simulink model "TCS_autosar_arch"  (R2019b)
settings: Solver=VariableStepAuto  StartTime=0.0  StopTime=10.0  RelTol=1e-3
settings Model: Creator=12045  LastModifiedBy=12045

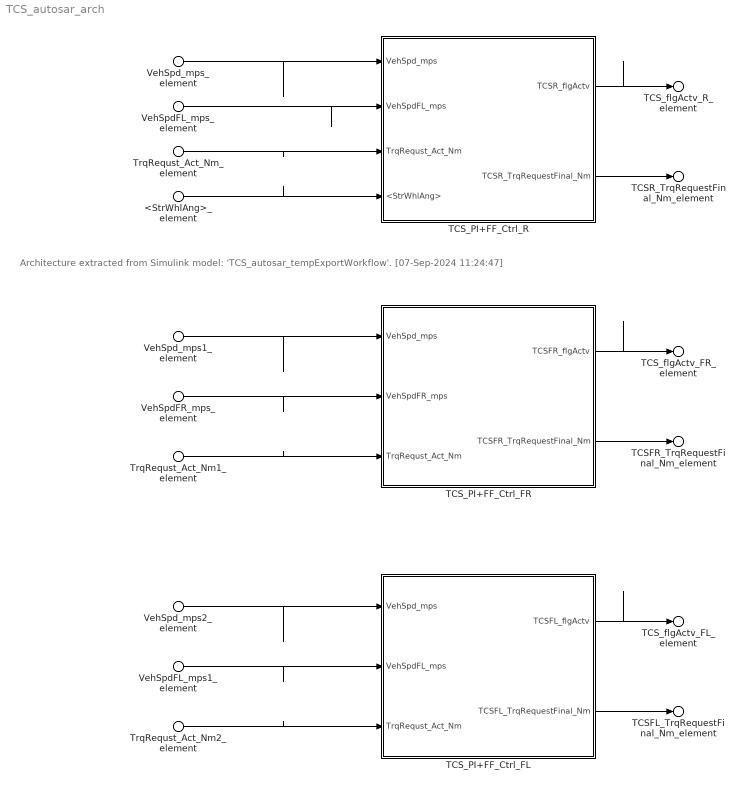
== system TCS_autosar_arch ==
  note: Architecture extracted from Simulink model: 'TCS_autosar_tempExportWorkflow'. [07-Sep-2024 11:24:47]
  VehSpd_mps_element : Inport  PortName=VehSpd_mps
  VehSpdFL_mps_element : Inport  Port=2  PortName=VehSpdFL_mps
  TrqRequst_Act_Nm_element : Inport  Port=3  PortName=TrqRequst_Act_Nm
  <StrWhlAng>_element : Inport  Port=4  PortName=<StrWhlAng>
  VehSpd_mps1_element : Inport  Port=5  PortName=VehSpd_mps1
  VehSpdFR_mps_element : Inport  Port=6  PortName=VehSpdFR_mps
  TrqRequst_Act_Nm1_element : Inport  Port=7  PortName=TrqRequst_Act_Nm1
  VehSpd_mps2_element : Inport  Port=8  PortName=VehSpd_mps2
  VehSpdFL_mps1_element : Inport  Port=9  PortName=VehSpdFL_mps1
  TrqRequst_Act_Nm2_element : Inport  Port=10  PortName=TrqRequst_Act_Nm2
  TCS_PI+FF_Ctrl_FL : Subsystem
      settings: PortSchema="{\"entries\":[{\"content\":{\"headerSize\":26,\"margin\":15,\"minimumSpacing\":25,\"sides\":[{\"content\":{\"connectorIds\":[\"In1\",\"In2\",\"In3\"]},\"type\":\"ConnectorPlacement.EquallySpacedRectSide\",\"uuid\":\"eaf1fc9b-c735-4d64-9f98-dd2769dd9966\"},{\"content\":{\"connectorIds\":[\"Out1\",\"Out2\"],\"side\":\"RIGHT\"},\"type\":\"ConnectorPlacement.EquallySpacedRectSide\",\"uuid\":\"44921fe4-cdee-42c2-ba14-46e851cbb056\"},{\"content\":{\"connectorIds\":[],\"side\":\"TOP\"},\"type\":\"ConnectorPlacement.EquallySpacedRectSide\",\"uuid\":\"3b219d8e-8c01-443b-b35e-1f0c6839a481\"}]},\"type\":\"ConnectorPlacement.EquallySpacedConnector\",\"uuid\":\"03372050-c4f7-4141-ad1c-5172546441aa\"}],\"packageUris\":[\"http://schema.mathworks.com/mf0/Connector/19700101\"],\"version\":\"1.0\"}"
  TCS_PI+FF_Ctrl_FR : Subsystem
      settings: PortSchema="{\"entries\":[{\"content\":{\"headerSize\":26,\"margin\":15,\"minimumSpacing\":25,\"sides\":[{\"content\":{\"connectorIds\":[\"In1\",\"In2\",\"In3\"]},\"type\":\"ConnectorPlacement.EquallySpacedRectSide\",\"uuid\":\"eaf1fc9b-c735-4d64-9f98-dd2769dd9966\"},{\"content\":{\"connectorIds\":[\"Out1\",\"Out2\"],\"side\":\"RIGHT\"},\"type\":\"ConnectorPlacement.EquallySpacedRectSide\",\"uuid\":\"44921fe4-cdee-42c2-ba14-46e851cbb056\"},{\"content\":{\"connectorIds\":[],\"side\":\"TOP\"},\"type\":\"ConnectorPlacement.EquallySpacedRectSide\",\"uuid\":\"3b219d8e-8c01-443b-b35e-1f0c6839a481\"}]},\"type\":\"ConnectorPlacement.EquallySpacedConnector\",\"uuid\":\"03372050-c4f7-4141-ad1c-5172546441aa\"}],\"packageUris\":[\"http://schema.mathworks.com/mf0/Connector/19700101\"],\"version\":\"1.0\"}"
  TCS_PI+FF_Ctrl_R : Subsystem
      settings: PortSchema="{\"entries\":[{\"content\":{\"headerSize\":26,\"margin\":15,\"minimumSpacing\":25,\"sides\":[{\"content\":{\"connectorIds\":[\"In1\",\"In2\",\"In3\",\"In4\"]},\"type\":\"ConnectorPlacement.EquallySpacedRectSide\",\"uuid\":\"eaf1fc9b-c735-4d64-9f98-dd2769dd9966\"},{\"content\":{\"connectorIds\":[\"Out1\",\"Out2\"],\"side\":\"RIGHT\"},\"type\":\"ConnectorPlacement.EquallySpacedRectSide\",\"uuid\":\"44921fe4-cdee-42c2-ba14-46e851cbb056\"},{\"content\":{\"connectorIds\":[],\"side\":\"TOP\"},\"type\":\"ConnectorPlacement.EquallySpacedRectSide\",\"uuid\":\"3b219d8e-8c01-443b-b35e-1f0c6839a481\"}]},\"type\":\"ConnectorPlacement.EquallySpacedConnector\",\"uuid\":\"03372050-c4f7-4141-ad1c-5172546441aa\"}],\"packageUris\":[\"http://schema.mathworks.com/mf0/Connector/19700101\"],\"version\":\"1.0\"}"
  TCS_flgActv_R_element : Outport  PortName=TCS_flgActv_R
  TCSR_TrqRequestFinal_Nm_element : Outport  Port=2  PortName=TCSR_TrqRequestFinal_Nm
  TCS_flgActv_FR_element : Outport  Port=3  PortName=TCS_flgActv_FR
  TCSFR_TrqRequestFinal_Nm_element : Outport  Port=4  PortName=TCSFR_TrqRequestFinal_Nm
  TCS_flgActv_FL_element : Outport  Port=5  PortName=TCS_flgActv_FL
  TCSFL_TrqRequestFinal_Nm_element : Outport  Port=6  PortName=TCSFL_TrqRequestFinal_Nm
  wires:
  VehSpd_mps2_element/1 -> TCS_PI+FF_Ctrl_FL/1(VehSpd_mps)
  VehSpdFL_mps1_element/1 -> TCS_PI+FF_Ctrl_FL/2(VehSpdFL_mps)
  TrqRequst_Act_Nm2_element/1 -> TCS_PI+FF_Ctrl_FL/3(TrqRequst_Act_Nm)
  VehSpd_mps1_element/1 -> TCS_PI+FF_Ctrl_FR/1(VehSpd_mps)
  VehSpdFR_mps_element/1 -> TCS_PI+FF_Ctrl_FR/2(VehSpdFR_mps)
  TrqRequst_Act_Nm1_element/1 -> TCS_PI+FF_Ctrl_FR/3(TrqRequst_Act_Nm)
  VehSpd_mps_element/1 -> TCS_PI+FF_Ctrl_R/1(VehSpd_mps)
  VehSpdFL_mps_element/1 -> TCS_PI+FF_Ctrl_R/2(VehSpdFL_mps)
  TrqRequst_Act_Nm_element/1 -> TCS_PI+FF_Ctrl_R/3(TrqRequst_Act_Nm)
  <StrWhlAng>_element/1 -> TCS_PI+FF_Ctrl_R/4(<StrWhlAng>)
  TCS_PI+FF_Ctrl_R/1(TCSR_flgActv) -> TCS_flgActv_R_element/1
  TCS_PI+FF_Ctrl_R/2(TCSR_TrqRequestFinal_Nm) -> TCSR_TrqRequestFinal_Nm_element/1
  TCS_PI+FF_Ctrl_FR/1(TCSFR_flgActv) -> TCS_flgActv_FR_element/1
  TCS_PI+FF_Ctrl_FR/2(TCSFR_TrqRequestFinal_Nm) -> TCSFR_TrqRequestFinal_Nm_element/1
  TCS_PI+FF_Ctrl_FL/1(TCSFL_flgActv) -> TCS_flgActv_FL_element/1
  TCS_PI+FF_Ctrl_FL/2(TCSFL_TrqRequestFinal_Nm) -> TCSFL_TrqRequestFinal_Nm_element/1

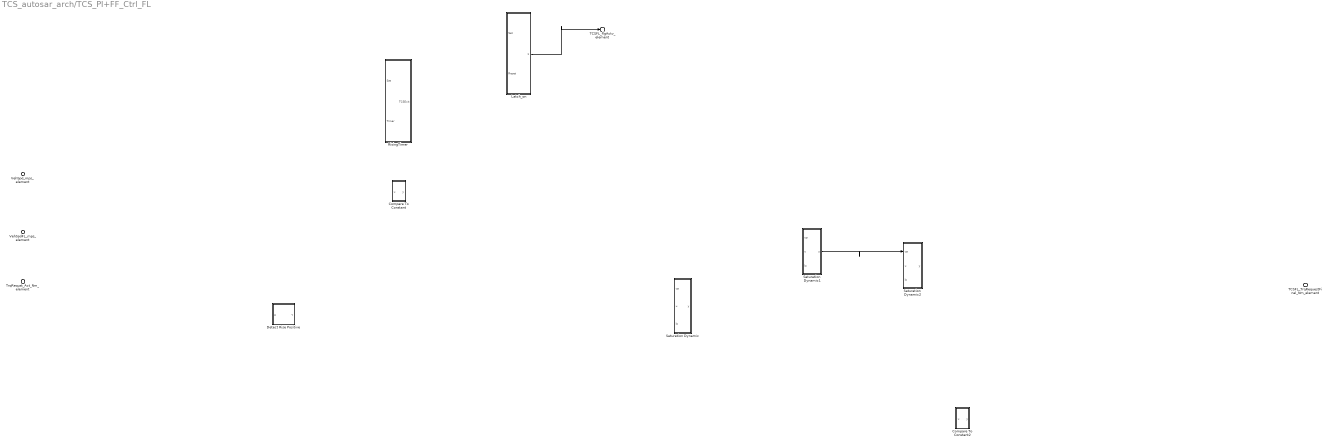
== system TCS_autosar_arch/TCS_PI+FF_Ctrl_FL ==
  VehSpd_mps_element : Inport  PortName=VehSpd_mps
  VehSpdFL_mps_element : Inport  Port=2  PortName=VehSpdFL_mps
  TrqRequst_Act_Nm_element : Inport  Port=3  PortName=TrqRequst_Act_Nm
  Compare To Constant : Subsystem
      settings: PortSchema="{\"entries\":[{\"content\":{\"headerSize\":26,\"margin\":15,\"minimumSpacing\":25,\"sides\":[{\"content\":{\"connectorIds\":[\"In1\"]},\"type\":\"ConnectorPlacement.EquallySpacedRectSide\",\"uuid\":\"eaf1fc9b-c735-4d64-9f98-dd2769dd9966\"},{\"content\":{\"connectorIds\":[\"Out1\"],\"side\":\"RIGHT\"},\"type\":\"ConnectorPlacement.EquallySpacedRectSide\",\"uuid\":\"44921fe4-cdee-42c2-ba14-46e851cbb056\"},{\"content\":{\"connectorIds\":[],\"side\":\"TOP\"},\"type\":\"ConnectorPlacement.EquallySpacedRectSide\",\"uuid\":\"3b219d8e-8c01-443b-b35e-1f0c6839a481\"}]},\"type\":\"ConnectorPlacement.EquallySpacedConnector\",\"uuid\":\"03372050-c4f7-4141-ad1c-5172546441aa\"}],\"packageUris\":[\"http://schema.mathworks.com/mf0/Connector/19700101\"],\"version\":\"1.0\"}"
  Compare To Constant2 : Subsystem
      settings: PortSchema="{\"entries\":[{\"content\":{\"headerSize\":26,\"margin\":15,\"minimumSpacing\":25,\"sides\":[{\"content\":{\"connectorIds\":[\"In1\"]},\"type\":\"ConnectorPlacement.EquallySpacedRectSide\",\"uuid\":\"eaf1fc9b-c735-4d64-9f98-dd2769dd9966\"},{\"content\":{\"connectorIds\":[\"Out1\"],\"side\":\"RIGHT\"},\"type\":\"ConnectorPlacement.EquallySpacedRectSide\",\"uuid\":\"44921fe4-cdee-42c2-ba14-46e851cbb056\"},{\"content\":{\"connectorIds\":[],\"side\":\"TOP\"},\"type\":\"ConnectorPlacement.EquallySpacedRectSide\",\"uuid\":\"3b219d8e-8c01-443b-b35e-1f0c6839a481\"}]},\"type\":\"ConnectorPlacement.EquallySpacedConnector\",\"uuid\":\"03372050-c4f7-4141-ad1c-5172546441aa\"}],\"packageUris\":[\"http://schema.mathworks.com/mf0/Connector/19700101\"],\"version\":\"1.0\"}"
  Detect Rise Positive : Subsystem
      settings: PortSchema="{\"entries\":[{\"content\":{\"headerSize\":26,\"margin\":15,\"minimumSpacing\":25,\"sides\":[{\"content\":{\"connectorIds\":[\"In1\"]},\"type\":\"ConnectorPlacement.EquallySpacedRectSide\",\"uuid\":\"eaf1fc9b-c735-4d64-9f98-dd2769dd9966\"},{\"content\":{\"connectorIds\":[\"Out1\"],\"side\":\"RIGHT\"},\"type\":\"ConnectorPlacement.EquallySpacedRectSide\",\"uuid\":\"44921fe4-cdee-42c2-ba14-46e851cbb056\"},{\"content\":{\"connectorIds\":[],\"side\":\"TOP\"},\"type\":\"ConnectorPlacement.EquallySpacedRectSide\",\"uuid\":\"3b219d8e-8c01-443b-b35e-1f0c6839a481\"}]},\"type\":\"ConnectorPlacement.EquallySpacedConnector\",\"uuid\":\"03372050-c4f7-4141-ad1c-5172546441aa\"}],\"packageUris\":[\"http://schema.mathworks.com/mf0/Connector/19700101\"],\"version\":\"1.0\"}"
  Latch_on : Subsystem
      settings: PortSchema="{\"entries\":[{\"content\":{\"headerSize\":26,\"margin\":15,\"minimumSpacing\":25,\"sides\":[{\"content\":{\"connectorIds\":[\"In1\",\"In2\"]},\"type\":\"ConnectorPlacement.EquallySpacedRectSide\",\"uuid\":\"eaf1fc9b-c735-4d64-9f98-dd2769dd9966\"},{\"content\":{\"connectorIds\":[\"Out1\"],\"side\":\"RIGHT\"},\"type\":\"ConnectorPlacement.EquallySpacedRectSide\",\"uuid\":\"44921fe4-cdee-42c2-ba14-46e851cbb056\"},{\"content\":{\"connectorIds\":[],\"side\":\"TOP\"},\"type\":\"ConnectorPlacement.EquallySpacedRectSide\",\"uuid\":\"3b219d8e-8c01-443b-b35e-1f0c6839a481\"}]},\"type\":\"ConnectorPlacement.EquallySpacedConnector\",\"uuid\":\"03372050-c4f7-4141-ad1c-5172546441aa\"}],\"packageUris\":[\"http://schema.mathworks.com/mf0/Connector/19700101\"],\"version\":\"1.0\"}"
  RisingTimer : Subsystem
      settings: PortSchema="{\"entries\":[{\"content\":{\"headerSize\":26,\"margin\":15,\"minimumSpacing\":25,\"sides\":[{\"content\":{\"connectorIds\":[\"In1\",\"In2\"]},\"type\":\"ConnectorPlacement.EquallySpacedRectSide\",\"uuid\":\"eaf1fc9b-c735-4d64-9f98-dd2769dd9966\"},{\"content\":{\"connectorIds\":[\"Out1\"],\"side\":\"RIGHT\"},\"type\":\"ConnectorPlacement.EquallySpacedRectSide\",\"uuid\":\"44921fe4-cdee-42c2-ba14-46e851cbb056\"},{\"content\":{\"connectorIds\":[],\"side\":\"TOP\"},\"type\":\"ConnectorPlacement.EquallySpacedRectSide\",\"uuid\":\"3b219d8e-8c01-443b-b35e-1f0c6839a481\"}]},\"type\":\"ConnectorPlacement.EquallySpacedConnector\",\"uuid\":\"03372050-c4f7-4141-ad1c-5172546441aa\"}],\"packageUris\":[\"http://schema.mathworks.com/mf0/Connector/19700101\"],\"version\":\"1.0\"}"
  Saturation Dynamic : Subsystem
      settings: PortSchema="{\"entries\":[{\"content\":{\"headerSize\":26,\"margin\":15,\"minimumSpacing\":25,\"sides\":[{\"content\":{\"connectorIds\":[\"In1\",\"In2\",\"In3\"]},\"type\":\"ConnectorPlacement.EquallySpacedRectSide\",\"uuid\":\"eaf1fc9b-c735-4d64-9f98-dd2769dd9966\"},{\"content\":{\"connectorIds\":[\"Out1\"],\"side\":\"RIGHT\"},\"type\":\"ConnectorPlacement.EquallySpacedRectSide\",\"uuid\":\"44921fe4-cdee-42c2-ba14-46e851cbb056\"},{\"content\":{\"connectorIds\":[],\"side\":\"TOP\"},\"type\":\"ConnectorPlacement.EquallySpacedRectSide\",\"uuid\":\"3b219d8e-8c01-443b-b35e-1f0c6839a481\"}]},\"type\":\"ConnectorPlacement.EquallySpacedConnector\",\"uuid\":\"03372050-c4f7-4141-ad1c-5172546441aa\"}],\"packageUris\":[\"http://schema.mathworks.com/mf0/Connector/19700101\"],\"version\":\"1.0\"}"
  Saturation Dynamic1 : Subsystem
      settings: PortSchema="{\"entries\":[{\"content\":{\"headerSize\":26,\"margin\":15,\"minimumSpacing\":25,\"sides\":[{\"content\":{\"connectorIds\":[\"In1\",\"In2\",\"In3\"]},\"type\":\"ConnectorPlacement.EquallySpacedRectSide\",\"uuid\":\"eaf1fc9b-c735-4d64-9f98-dd2769dd9966\"},{\"content\":{\"connectorIds\":[\"Out1\"],\"side\":\"RIGHT\"},\"type\":\"ConnectorPlacement.EquallySpacedRectSide\",\"uuid\":\"44921fe4-cdee-42c2-ba14-46e851cbb056\"},{\"content\":{\"connectorIds\":[],\"side\":\"TOP\"},\"type\":\"ConnectorPlacement.EquallySpacedRectSide\",\"uuid\":\"3b219d8e-8c01-443b-b35e-1f0c6839a481\"}]},\"type\":\"ConnectorPlacement.EquallySpacedConnector\",\"uuid\":\"03372050-c4f7-4141-ad1c-5172546441aa\"}],\"packageUris\":[\"http://schema.mathworks.com/mf0/Connector/19700101\"],\"version\":\"1.0\"}"
  Saturation Dynamic2 : Subsystem
      settings: PortSchema="{\"entries\":[{\"content\":{\"headerSize\":26,\"margin\":15,\"minimumSpacing\":25,\"sides\":[{\"content\":{\"connectorIds\":[\"In1\",\"In2\",\"In3\"]},\"type\":\"ConnectorPlacement.EquallySpacedRectSide\",\"uuid\":\"eaf1fc9b-c735-4d64-9f98-dd2769dd9966\"},{\"content\":{\"connectorIds\":[\"Out1\"],\"side\":\"RIGHT\"},\"type\":\"ConnectorPlacement.EquallySpacedRectSide\",\"uuid\":\"44921fe4-cdee-42c2-ba14-46e851cbb056\"},{\"content\":{\"connectorIds\":[],\"side\":\"TOP\"},\"type\":\"ConnectorPlacement.EquallySpacedRectSide\",\"uuid\":\"3b219d8e-8c01-443b-b35e-1f0c6839a481\"}]},\"type\":\"ConnectorPlacement.EquallySpacedConnector\",\"uuid\":\"03372050-c4f7-4141-ad1c-5172546441aa\"}],\"packageUris\":[\"http://schema.mathworks.com/mf0/Connector/19700101\"],\"version\":\"1.0\"}"
  TCSFL_flgActv_element : Outport  PortName=TCSFL_flgActv
  TCSFL_TrqRequestFinal_Nm_element : Outport  Port=2  PortName=TCSFL_TrqRequestFinal_Nm
  wires:
  Saturation Dynamic1/1(y) -> Saturation Dynamic2/1(up)
  Latch_on/1(flg_TCSActv) -> TCSFL_flgActv_element/1

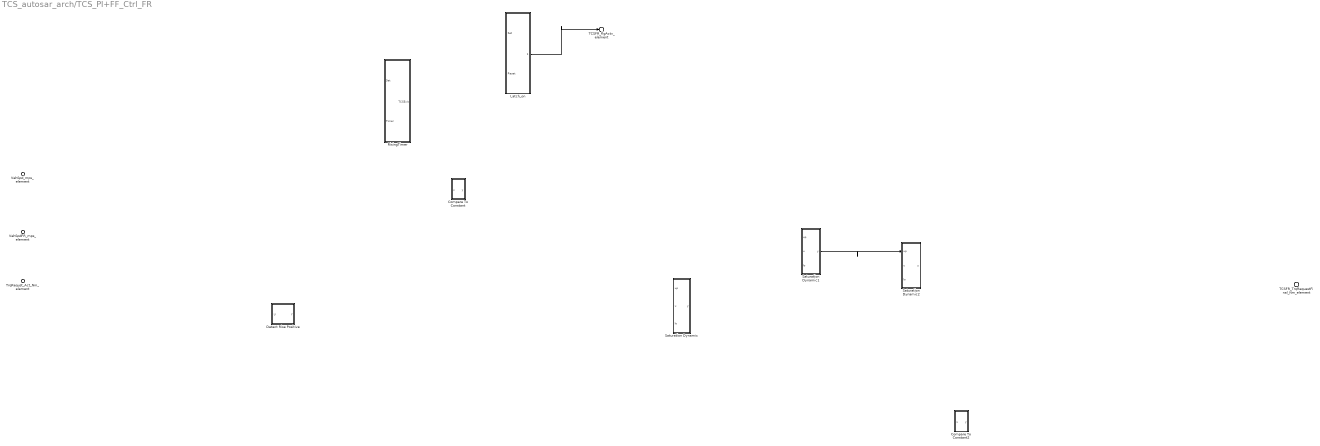
== system TCS_autosar_arch/TCS_PI+FF_Ctrl_FR ==
  VehSpd_mps_element : Inport  PortName=VehSpd_mps
  VehSpdFR_mps_element : Inport  Port=2  PortName=VehSpdFR_mps
  TrqRequst_Act_Nm_element : Inport  Port=3  PortName=TrqRequst_Act_Nm
  Compare To Constant : Subsystem
      settings: PortSchema="{\"entries\":[{\"content\":{\"headerSize\":26,\"margin\":15,\"minimumSpacing\":25,\"sides\":[{\"content\":{\"connectorIds\":[\"In1\"]},\"type\":\"ConnectorPlacement.EquallySpacedRectSide\",\"uuid\":\"eaf1fc9b-c735-4d64-9f98-dd2769dd9966\"},{\"content\":{\"connectorIds\":[\"Out1\"],\"side\":\"RIGHT\"},\"type\":\"ConnectorPlacement.EquallySpacedRectSide\",\"uuid\":\"44921fe4-cdee-42c2-ba14-46e851cbb056\"},{\"content\":{\"connectorIds\":[],\"side\":\"TOP\"},\"type\":\"ConnectorPlacement.EquallySpacedRectSide\",\"uuid\":\"3b219d8e-8c01-443b-b35e-1f0c6839a481\"}]},\"type\":\"ConnectorPlacement.EquallySpacedConnector\",\"uuid\":\"03372050-c4f7-4141-ad1c-5172546441aa\"}],\"packageUris\":[\"http://schema.mathworks.com/mf0/Connector/19700101\"],\"version\":\"1.0\"}"
  Compare To Constant2 : Subsystem
      settings: PortSchema="{\"entries\":[{\"content\":{\"headerSize\":26,\"margin\":15,\"minimumSpacing\":25,\"sides\":[{\"content\":{\"connectorIds\":[\"In1\"]},\"type\":\"ConnectorPlacement.EquallySpacedRectSide\",\"uuid\":\"eaf1fc9b-c735-4d64-9f98-dd2769dd9966\"},{\"content\":{\"connectorIds\":[\"Out1\"],\"side\":\"RIGHT\"},\"type\":\"ConnectorPlacement.EquallySpacedRectSide\",\"uuid\":\"44921fe4-cdee-42c2-ba14-46e851cbb056\"},{\"content\":{\"connectorIds\":[],\"side\":\"TOP\"},\"type\":\"ConnectorPlacement.EquallySpacedRectSide\",\"uuid\":\"3b219d8e-8c01-443b-b35e-1f0c6839a481\"}]},\"type\":\"ConnectorPlacement.EquallySpacedConnector\",\"uuid\":\"03372050-c4f7-4141-ad1c-5172546441aa\"}],\"packageUris\":[\"http://schema.mathworks.com/mf0/Connector/19700101\"],\"version\":\"1.0\"}"
  Detect Rise Positive : Subsystem
      settings: PortSchema="{\"entries\":[{\"content\":{\"headerSize\":26,\"margin\":15,\"minimumSpacing\":25,\"sides\":[{\"content\":{\"connectorIds\":[\"In1\"]},\"type\":\"ConnectorPlacement.EquallySpacedRectSide\",\"uuid\":\"eaf1fc9b-c735-4d64-9f98-dd2769dd9966\"},{\"content\":{\"connectorIds\":[\"Out1\"],\"side\":\"RIGHT\"},\"type\":\"ConnectorPlacement.EquallySpacedRectSide\",\"uuid\":\"44921fe4-cdee-42c2-ba14-46e851cbb056\"},{\"content\":{\"connectorIds\":[],\"side\":\"TOP\"},\"type\":\"ConnectorPlacement.EquallySpacedRectSide\",\"uuid\":\"3b219d8e-8c01-443b-b35e-1f0c6839a481\"}]},\"type\":\"ConnectorPlacement.EquallySpacedConnector\",\"uuid\":\"03372050-c4f7-4141-ad1c-5172546441aa\"}],\"packageUris\":[\"http://schema.mathworks.com/mf0/Connector/19700101\"],\"version\":\"1.0\"}"
  Latch_on : Subsystem
      settings: PortSchema="{\"entries\":[{\"content\":{\"headerSize\":26,\"margin\":15,\"minimumSpacing\":25,\"sides\":[{\"content\":{\"connectorIds\":[\"In1\",\"In2\"]},\"type\":\"ConnectorPlacement.EquallySpacedRectSide\",\"uuid\":\"eaf1fc9b-c735-4d64-9f98-dd2769dd9966\"},{\"content\":{\"connectorIds\":[\"Out1\"],\"side\":\"RIGHT\"},\"type\":\"ConnectorPlacement.EquallySpacedRectSide\",\"uuid\":\"44921fe4-cdee-42c2-ba14-46e851cbb056\"},{\"content\":{\"connectorIds\":[],\"side\":\"TOP\"},\"type\":\"ConnectorPlacement.EquallySpacedRectSide\",\"uuid\":\"3b219d8e-8c01-443b-b35e-1f0c6839a481\"}]},\"type\":\"ConnectorPlacement.EquallySpacedConnector\",\"uuid\":\"03372050-c4f7-4141-ad1c-5172546441aa\"}],\"packageUris\":[\"http://schema.mathworks.com/mf0/Connector/19700101\"],\"version\":\"1.0\"}"
  RisingTimer : Subsystem
      settings: PortSchema="{\"entries\":[{\"content\":{\"headerSize\":26,\"margin\":15,\"minimumSpacing\":25,\"sides\":[{\"content\":{\"connectorIds\":[\"In1\",\"In2\"]},\"type\":\"ConnectorPlacement.EquallySpacedRectSide\",\"uuid\":\"eaf1fc9b-c735-4d64-9f98-dd2769dd9966\"},{\"content\":{\"connectorIds\":[\"Out1\"],\"side\":\"RIGHT\"},\"type\":\"ConnectorPlacement.EquallySpacedRectSide\",\"uuid\":\"44921fe4-cdee-42c2-ba14-46e851cbb056\"},{\"content\":{\"connectorIds\":[],\"side\":\"TOP\"},\"type\":\"ConnectorPlacement.EquallySpacedRectSide\",\"uuid\":\"3b219d8e-8c01-443b-b35e-1f0c6839a481\"}]},\"type\":\"ConnectorPlacement.EquallySpacedConnector\",\"uuid\":\"03372050-c4f7-4141-ad1c-5172546441aa\"}],\"packageUris\":[\"http://schema.mathworks.com/mf0/Connector/19700101\"],\"version\":\"1.0\"}"
  Saturation Dynamic : Subsystem
      settings: PortSchema="{\"entries\":[{\"content\":{\"headerSize\":26,\"margin\":15,\"minimumSpacing\":25,\"sides\":[{\"content\":{\"connectorIds\":[\"In1\",\"In2\",\"In3\"]},\"type\":\"ConnectorPlacement.EquallySpacedRectSide\",\"uuid\":\"eaf1fc9b-c735-4d64-9f98-dd2769dd9966\"},{\"content\":{\"connectorIds\":[\"Out1\"],\"side\":\"RIGHT\"},\"type\":\"ConnectorPlacement.EquallySpacedRectSide\",\"uuid\":\"44921fe4-cdee-42c2-ba14-46e851cbb056\"},{\"content\":{\"connectorIds\":[],\"side\":\"TOP\"},\"type\":\"ConnectorPlacement.EquallySpacedRectSide\",\"uuid\":\"3b219d8e-8c01-443b-b35e-1f0c6839a481\"}]},\"type\":\"ConnectorPlacement.EquallySpacedConnector\",\"uuid\":\"03372050-c4f7-4141-ad1c-5172546441aa\"}],\"packageUris\":[\"http://schema.mathworks.com/mf0/Connector/19700101\"],\"version\":\"1.0\"}"
  Saturation Dynamic1 : Subsystem
      settings: PortSchema="{\"entries\":[{\"content\":{\"headerSize\":26,\"margin\":15,\"minimumSpacing\":25,\"sides\":[{\"content\":{\"connectorIds\":[\"In1\",\"In2\",\"In3\"]},\"type\":\"ConnectorPlacement.EquallySpacedRectSide\",\"uuid\":\"eaf1fc9b-c735-4d64-9f98-dd2769dd9966\"},{\"content\":{\"connectorIds\":[\"Out1\"],\"side\":\"RIGHT\"},\"type\":\"ConnectorPlacement.EquallySpacedRectSide\",\"uuid\":\"44921fe4-cdee-42c2-ba14-46e851cbb056\"},{\"content\":{\"connectorIds\":[],\"side\":\"TOP\"},\"type\":\"ConnectorPlacement.EquallySpacedRectSide\",\"uuid\":\"3b219d8e-8c01-443b-b35e-1f0c6839a481\"}]},\"type\":\"ConnectorPlacement.EquallySpacedConnector\",\"uuid\":\"03372050-c4f7-4141-ad1c-5172546441aa\"}],\"packageUris\":[\"http://schema.mathworks.com/mf0/Connector/19700101\"],\"version\":\"1.0\"}"
  Saturation Dynamic2 : Subsystem
      settings: PortSchema="{\"entries\":[{\"content\":{\"headerSize\":26,\"margin\":15,\"minimumSpacing\":25,\"sides\":[{\"content\":{\"connectorIds\":[\"In1\",\"In2\",\"In3\"]},\"type\":\"ConnectorPlacement.EquallySpacedRectSide\",\"uuid\":\"eaf1fc9b-c735-4d64-9f98-dd2769dd9966\"},{\"content\":{\"connectorIds\":[\"Out1\"],\"side\":\"RIGHT\"},\"type\":\"ConnectorPlacement.EquallySpacedRectSide\",\"uuid\":\"44921fe4-cdee-42c2-ba14-46e851cbb056\"},{\"content\":{\"connectorIds\":[],\"side\":\"TOP\"},\"type\":\"ConnectorPlacement.EquallySpacedRectSide\",\"uuid\":\"3b219d8e-8c01-443b-b35e-1f0c6839a481\"}]},\"type\":\"ConnectorPlacement.EquallySpacedConnector\",\"uuid\":\"03372050-c4f7-4141-ad1c-5172546441aa\"}],\"packageUris\":[\"http://schema.mathworks.com/mf0/Connector/19700101\"],\"version\":\"1.0\"}"
  TCSFR_flgActv_element : Outport  PortName=TCSFR_flgActv
  TCSFR_TrqRequestFinal_Nm_element : Outport  Port=2  PortName=TCSFR_TrqRequestFinal_Nm
  wires:
  Saturation Dynamic1/1(y) -> Saturation Dynamic2/1(up)
  Latch_on/1(flg_TCSActv) -> TCSFR_flgActv_element/1

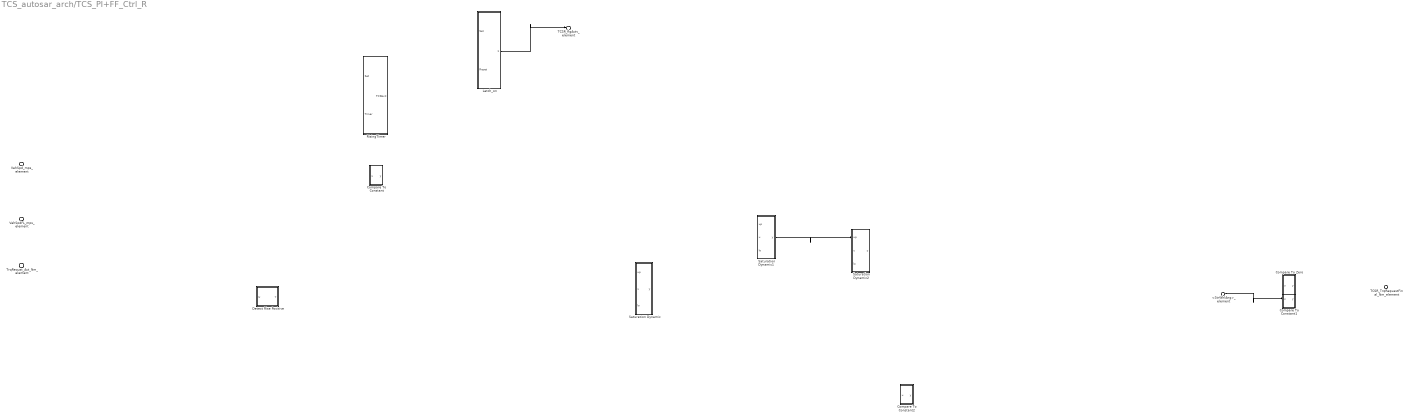
== system TCS_autosar_arch/TCS_PI+FF_Ctrl_R ==
  VehSpd_mps_element : Inport  PortName=VehSpd_mps
  VehSpdFL_mps_element : Inport  Port=2  PortName=VehSpdFL_mps
  TrqRequst_Act_Nm_element : Inport  Port=3  PortName=TrqRequst_Act_Nm
  <StrWhlAng>_element : Inport  Port=4  PortName=<StrWhlAng>
  Compare To Constant : Subsystem
      settings: PortSchema="{\"entries\":[{\"content\":{\"headerSize\":26,\"margin\":15,\"minimumSpacing\":25,\"sides\":[{\"content\":{\"connectorIds\":[\"In1\"]},\"type\":\"ConnectorPlacement.EquallySpacedRectSide\",\"uuid\":\"eaf1fc9b-c735-4d64-9f98-dd2769dd9966\"},{\"content\":{\"connectorIds\":[\"Out1\"],\"side\":\"RIGHT\"},\"type\":\"ConnectorPlacement.EquallySpacedRectSide\",\"uuid\":\"44921fe4-cdee-42c2-ba14-46e851cbb056\"},{\"content\":{\"connectorIds\":[],\"side\":\"TOP\"},\"type\":\"ConnectorPlacement.EquallySpacedRectSide\",\"uuid\":\"3b219d8e-8c01-443b-b35e-1f0c6839a481\"}]},\"type\":\"ConnectorPlacement.EquallySpacedConnector\",\"uuid\":\"03372050-c4f7-4141-ad1c-5172546441aa\"}],\"packageUris\":[\"http://schema.mathworks.com/mf0/Connector/19700101\"],\"version\":\"1.0\"}"
  Compare To Constant1 : Subsystem
      settings: PortSchema="{\"entries\":[{\"content\":{\"headerSize\":26,\"margin\":15,\"minimumSpacing\":25,\"sides\":[{\"content\":{\"connectorIds\":[\"In1\"]},\"type\":\"ConnectorPlacement.EquallySpacedRectSide\",\"uuid\":\"eaf1fc9b-c735-4d64-9f98-dd2769dd9966\"},{\"content\":{\"connectorIds\":[\"Out1\"],\"side\":\"RIGHT\"},\"type\":\"ConnectorPlacement.EquallySpacedRectSide\",\"uuid\":\"44921fe4-cdee-42c2-ba14-46e851cbb056\"},{\"content\":{\"connectorIds\":[],\"side\":\"TOP\"},\"type\":\"ConnectorPlacement.EquallySpacedRectSide\",\"uuid\":\"3b219d8e-8c01-443b-b35e-1f0c6839a481\"}]},\"type\":\"ConnectorPlacement.EquallySpacedConnector\",\"uuid\":\"03372050-c4f7-4141-ad1c-5172546441aa\"}],\"packageUris\":[\"http://schema.mathworks.com/mf0/Connector/19700101\"],\"version\":\"1.0\"}"
  Compare To Constant2 : Subsystem
      settings: PortSchema="{\"entries\":[{\"content\":{\"headerSize\":26,\"margin\":15,\"minimumSpacing\":25,\"sides\":[{\"content\":{\"connectorIds\":[\"In1\"]},\"type\":\"ConnectorPlacement.EquallySpacedRectSide\",\"uuid\":\"eaf1fc9b-c735-4d64-9f98-dd2769dd9966\"},{\"content\":{\"connectorIds\":[\"Out1\"],\"side\":\"RIGHT\"},\"type\":\"ConnectorPlacement.EquallySpacedRectSide\",\"uuid\":\"44921fe4-cdee-42c2-ba14-46e851cbb056\"},{\"content\":{\"connectorIds\":[],\"side\":\"TOP\"},\"type\":\"ConnectorPlacement.EquallySpacedRectSide\",\"uuid\":\"3b219d8e-8c01-443b-b35e-1f0c6839a481\"}]},\"type\":\"ConnectorPlacement.EquallySpacedConnector\",\"uuid\":\"03372050-c4f7-4141-ad1c-5172546441aa\"}],\"packageUris\":[\"http://schema.mathworks.com/mf0/Connector/19700101\"],\"version\":\"1.0\"}"
  Compare To Zero : Subsystem
      settings: PortSchema="{\"entries\":[{\"content\":{\"headerSize\":26,\"margin\":15,\"minimumSpacing\":25,\"sides\":[{\"content\":{\"connectorIds\":[\"In1\"]},\"type\":\"ConnectorPlacement.EquallySpacedRectSide\",\"uuid\":\"eaf1fc9b-c735-4d64-9f98-dd2769dd9966\"},{\"content\":{\"connectorIds\":[\"Out1\"],\"side\":\"RIGHT\"},\"type\":\"ConnectorPlacement.EquallySpacedRectSide\",\"uuid\":\"44921fe4-cdee-42c2-ba14-46e851cbb056\"},{\"content\":{\"connectorIds\":[],\"side\":\"TOP\"},\"type\":\"ConnectorPlacement.EquallySpacedRectSide\",\"uuid\":\"3b219d8e-8c01-443b-b35e-1f0c6839a481\"}]},\"type\":\"ConnectorPlacement.EquallySpacedConnector\",\"uuid\":\"03372050-c4f7-4141-ad1c-5172546441aa\"}],\"packageUris\":[\"http://schema.mathworks.com/mf0/Connector/19700101\"],\"version\":\"1.0\"}"
  Detect Rise Positive : Subsystem
      settings: PortSchema="{\"entries\":[{\"content\":{\"headerSize\":26,\"margin\":15,\"minimumSpacing\":25,\"sides\":[{\"content\":{\"connectorIds\":[\"In1\"]},\"type\":\"ConnectorPlacement.EquallySpacedRectSide\",\"uuid\":\"eaf1fc9b-c735-4d64-9f98-dd2769dd9966\"},{\"content\":{\"connectorIds\":[\"Out1\"],\"side\":\"RIGHT\"},\"type\":\"ConnectorPlacement.EquallySpacedRectSide\",\"uuid\":\"44921fe4-cdee-42c2-ba14-46e851cbb056\"},{\"content\":{\"connectorIds\":[],\"side\":\"TOP\"},\"type\":\"ConnectorPlacement.EquallySpacedRectSide\",\"uuid\":\"3b219d8e-8c01-443b-b35e-1f0c6839a481\"}]},\"type\":\"ConnectorPlacement.EquallySpacedConnector\",\"uuid\":\"03372050-c4f7-4141-ad1c-5172546441aa\"}],\"packageUris\":[\"http://schema.mathworks.com/mf0/Connector/19700101\"],\"version\":\"1.0\"}"
  Latch_on : Subsystem
      settings: PortSchema="{\"entries\":[{\"content\":{\"headerSize\":26,\"margin\":15,\"minimumSpacing\":25,\"sides\":[{\"content\":{\"connectorIds\":[\"In1\",\"In2\"]},\"type\":\"ConnectorPlacement.EquallySpacedRectSide\",\"uuid\":\"eaf1fc9b-c735-4d64-9f98-dd2769dd9966\"},{\"content\":{\"connectorIds\":[\"Out1\"],\"side\":\"RIGHT\"},\"type\":\"ConnectorPlacement.EquallySpacedRectSide\",\"uuid\":\"44921fe4-cdee-42c2-ba14-46e851cbb056\"},{\"content\":{\"connectorIds\":[],\"side\":\"TOP\"},\"type\":\"ConnectorPlacement.EquallySpacedRectSide\",\"uuid\":\"3b219d8e-8c01-443b-b35e-1f0c6839a481\"}]},\"type\":\"ConnectorPlacement.EquallySpacedConnector\",\"uuid\":\"03372050-c4f7-4141-ad1c-5172546441aa\"}],\"packageUris\":[\"http://schema.mathworks.com/mf0/Connector/19700101\"],\"version\":\"1.0\"}"
  RisingTimer : Subsystem
      settings: PortSchema="{\"entries\":[{\"content\":{\"headerSize\":26,\"margin\":15,\"minimumSpacing\":25,\"sides\":[{\"content\":{\"connectorIds\":[\"In1\",\"In2\"]},\"type\":\"ConnectorPlacement.EquallySpacedRectSide\",\"uuid\":\"eaf1fc9b-c735-4d64-9f98-dd2769dd9966\"},{\"content\":{\"connectorIds\":[\"Out1\"],\"side\":\"RIGHT\"},\"type\":\"ConnectorPlacement.EquallySpacedRectSide\",\"uuid\":\"44921fe4-cdee-42c2-ba14-46e851cbb056\"},{\"content\":{\"connectorIds\":[],\"side\":\"TOP\"},\"type\":\"ConnectorPlacement.EquallySpacedRectSide\",\"uuid\":\"3b219d8e-8c01-443b-b35e-1f0c6839a481\"}]},\"type\":\"ConnectorPlacement.EquallySpacedConnector\",\"uuid\":\"03372050-c4f7-4141-ad1c-5172546441aa\"}],\"packageUris\":[\"http://schema.mathworks.com/mf0/Connector/19700101\"],\"version\":\"1.0\"}"
  Saturation Dynamic : Subsystem
      settings: PortSchema="{\"entries\":[{\"content\":{\"headerSize\":26,\"margin\":15,\"minimumSpacing\":25,\"sides\":[{\"content\":{\"connectorIds\":[\"In1\",\"In2\",\"In3\"]},\"type\":\"ConnectorPlacement.EquallySpacedRectSide\",\"uuid\":\"eaf1fc9b-c735-4d64-9f98-dd2769dd9966\"},{\"content\":{\"connectorIds\":[\"Out1\"],\"side\":\"RIGHT\"},\"type\":\"ConnectorPlacement.EquallySpacedRectSide\",\"uuid\":\"44921fe4-cdee-42c2-ba14-46e851cbb056\"},{\"content\":{\"connectorIds\":[],\"side\":\"TOP\"},\"type\":\"ConnectorPlacement.EquallySpacedRectSide\",\"uuid\":\"3b219d8e-8c01-443b-b35e-1f0c6839a481\"}]},\"type\":\"ConnectorPlacement.EquallySpacedConnector\",\"uuid\":\"03372050-c4f7-4141-ad1c-5172546441aa\"}],\"packageUris\":[\"http://schema.mathworks.com/mf0/Connector/19700101\"],\"version\":\"1.0\"}"
  Saturation Dynamic1 : Subsystem
      settings: PortSchema="{\"entries\":[{\"content\":{\"headerSize\":26,\"margin\":15,\"minimumSpacing\":25,\"sides\":[{\"content\":{\"connectorIds\":[\"In1\",\"In2\",\"In3\"]},\"type\":\"ConnectorPlacement.EquallySpacedRectSide\",\"uuid\":\"eaf1fc9b-c735-4d64-9f98-dd2769dd9966\"},{\"content\":{\"connectorIds\":[\"Out1\"],\"side\":\"RIGHT\"},\"type\":\"ConnectorPlacement.EquallySpacedRectSide\",\"uuid\":\"44921fe4-cdee-42c2-ba14-46e851cbb056\"},{\"content\":{\"connectorIds\":[],\"side\":\"TOP\"},\"type\":\"ConnectorPlacement.EquallySpacedRectSide\",\"uuid\":\"3b219d8e-8c01-443b-b35e-1f0c6839a481\"}]},\"type\":\"ConnectorPlacement.EquallySpacedConnector\",\"uuid\":\"03372050-c4f7-4141-ad1c-5172546441aa\"}],\"packageUris\":[\"http://schema.mathworks.com/mf0/Connector/19700101\"],\"version\":\"1.0\"}"
  Saturation Dynamic2 : Subsystem
      settings: PortSchema="{\"entries\":[{\"content\":{\"headerSize\":26,\"margin\":15,\"minimumSpacing\":25,\"sides\":[{\"content\":{\"connectorIds\":[\"In1\",\"In2\",\"In3\"]},\"type\":\"ConnectorPlacement.EquallySpacedRectSide\",\"uuid\":\"eaf1fc9b-c735-4d64-9f98-dd2769dd9966\"},{\"content\":{\"connectorIds\":[\"Out1\"],\"side\":\"RIGHT\"},\"type\":\"ConnectorPlacement.EquallySpacedRectSide\",\"uuid\":\"44921fe4-cdee-42c2-ba14-46e851cbb056\"},{\"content\":{\"connectorIds\":[],\"side\":\"TOP\"},\"type\":\"ConnectorPlacement.EquallySpacedRectSide\",\"uuid\":\"3b219d8e-8c01-443b-b35e-1f0c6839a481\"}]},\"type\":\"ConnectorPlacement.EquallySpacedConnector\",\"uuid\":\"03372050-c4f7-4141-ad1c-5172546441aa\"}],\"packageUris\":[\"http://schema.mathworks.com/mf0/Connector/19700101\"],\"version\":\"1.0\"}"
  TCSR_flgActv_element : Outport  PortName=TCSR_flgActv
  TCSR_TrqRequestFinal_Nm_element : Outport  Port=2  PortName=TCSR_TrqRequestFinal_Nm
  wires:
  <StrWhlAng>_element/1 -> Compare To Constant1/1(u)
  Saturation Dynamic1/1(y) -> Saturation Dynamic2/1(up)
  Latch_on/1(flg_TCSActv) -> TCSR_flgActv_element/1

== system TCS_autosar_arch/TCS_PI+FF_Ctrl_FL/Compare To Constant ==
  u_element : Inport  PortName=u
  y_element : Outport  PortName=y

== system TCS_autosar_arch/TCS_PI+FF_Ctrl_FL/Compare To Constant2 ==
  u_element : Inport  PortName=u
  y_element : Outport  PortName=y

== system TCS_autosar_arch/TCS_PI+FF_Ctrl_FL/Detect Rise Positive ==
  U_element : Inport  PortName=U
  Y_element : Outport  PortName=Y

== system TCS_autosar_arch/TCS_PI+FF_Ctrl_FL/Latch_on ==
  Set_element : Inport  PortName=Set
  Reset_element : Inport  Port=2  PortName=Reset
  flg_TCSActv_element : Outport  PortName=flg_TCSActv

== system TCS_autosar_arch/TCS_PI+FF_Ctrl_FL/RisingTimer ==
  Set_element : Inport  PortName=Set
  Timer_element : Inport  Port=2  PortName=Timer
  TCSExit_element : Outport  PortName=TCSExit

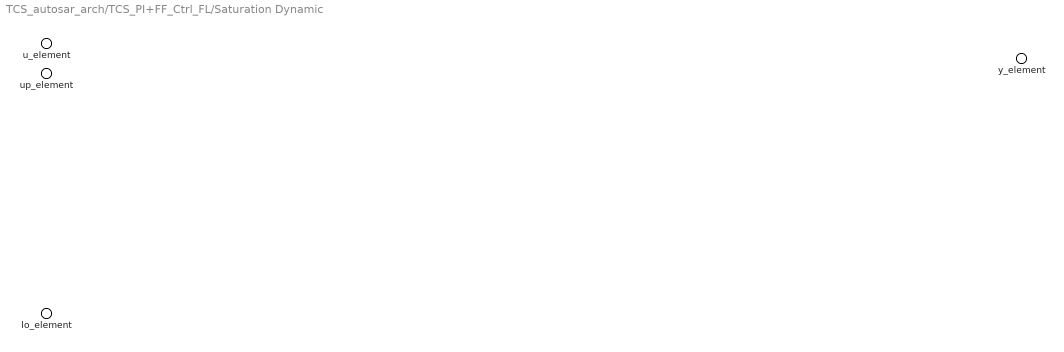
== system TCS_autosar_arch/TCS_PI+FF_Ctrl_FL/Saturation Dynamic ==
  up_element : Inport  PortName=up
  u_element : Inport  Port=2  PortName=u
  lo_element : Inport  Port=3  PortName=lo
  y_element : Outport  PortName=y

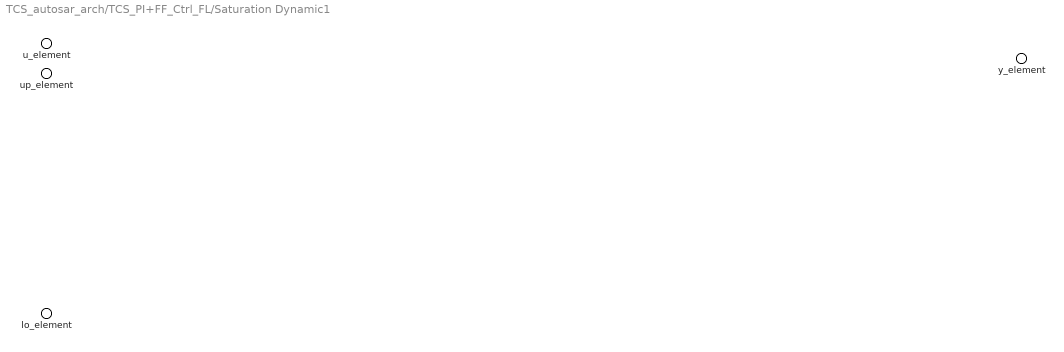
== system TCS_autosar_arch/TCS_PI+FF_Ctrl_FL/Saturation Dynamic1 ==
  up_element : Inport  PortName=up
  u_element : Inport  Port=2  PortName=u
  lo_element : Inport  Port=3  PortName=lo
  y_element : Outport  PortName=y

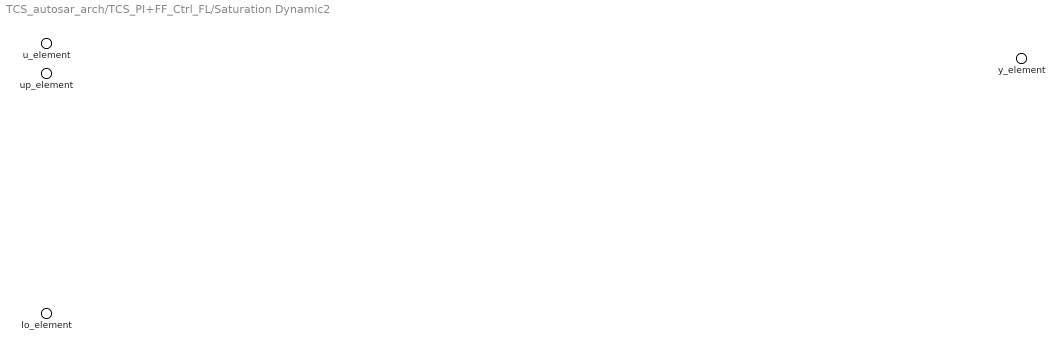
== system TCS_autosar_arch/TCS_PI+FF_Ctrl_FL/Saturation Dynamic2 ==
  up_element : Inport  PortName=up
  u_element : Inport  Port=2  PortName=u
  lo_element : Inport  Port=3  PortName=lo
  y_element : Outport  PortName=y

== system TCS_autosar_arch/TCS_PI+FF_Ctrl_FR/Compare To Constant ==
  u_element : Inport  PortName=u
  y_element : Outport  PortName=y

== system TCS_autosar_arch/TCS_PI+FF_Ctrl_FR/Compare To Constant2 ==
  u_element : Inport  PortName=u
  y_element : Outport  PortName=y

== system TCS_autosar_arch/TCS_PI+FF_Ctrl_FR/Detect Rise Positive ==
  U_element : Inport  PortName=U
  Y_element : Outport  PortName=Y

== system TCS_autosar_arch/TCS_PI+FF_Ctrl_FR/Latch_on ==
  Set_element : Inport  PortName=Set
  Reset_element : Inport  Port=2  PortName=Reset
  flg_TCSActv_element : Outport  PortName=flg_TCSActv

== system TCS_autosar_arch/TCS_PI+FF_Ctrl_FR/RisingTimer ==
  Set_element : Inport  PortName=Set
  Timer_element : Inport  Port=2  PortName=Timer
  TCSExit_element : Outport  PortName=TCSExit

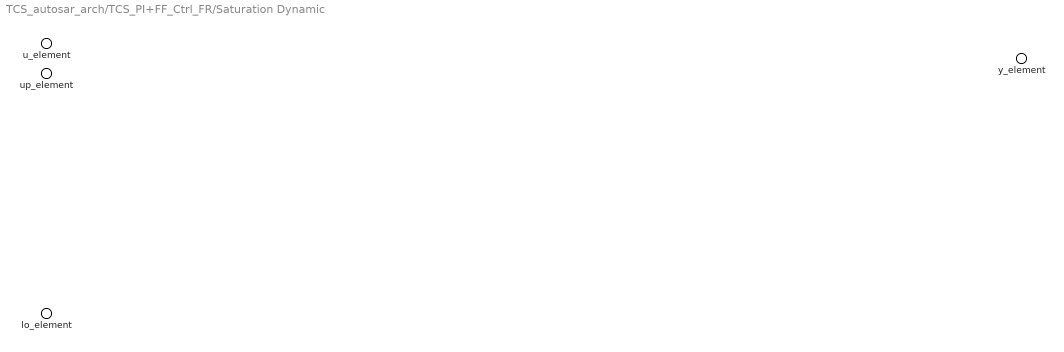
== system TCS_autosar_arch/TCS_PI+FF_Ctrl_FR/Saturation Dynamic ==
  up_element : Inport  PortName=up
  u_element : Inport  Port=2  PortName=u
  lo_element : Inport  Port=3  PortName=lo
  y_element : Outport  PortName=y

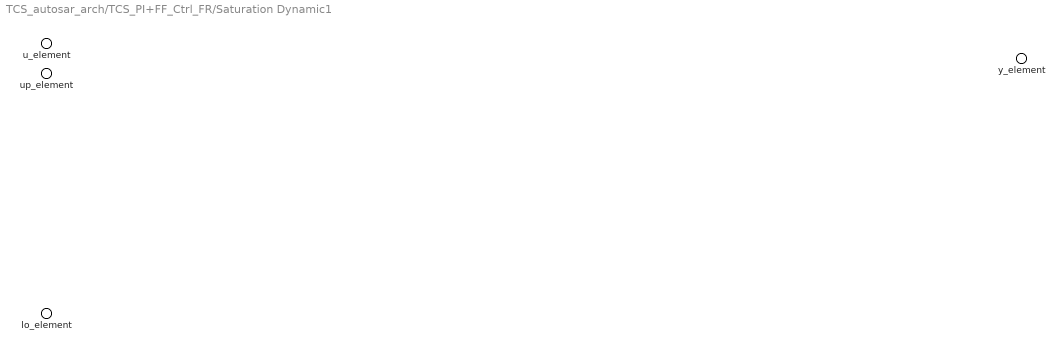
== system TCS_autosar_arch/TCS_PI+FF_Ctrl_FR/Saturation Dynamic1 ==
  up_element : Inport  PortName=up
  u_element : Inport  Port=2  PortName=u
  lo_element : Inport  Port=3  PortName=lo
  y_element : Outport  PortName=y

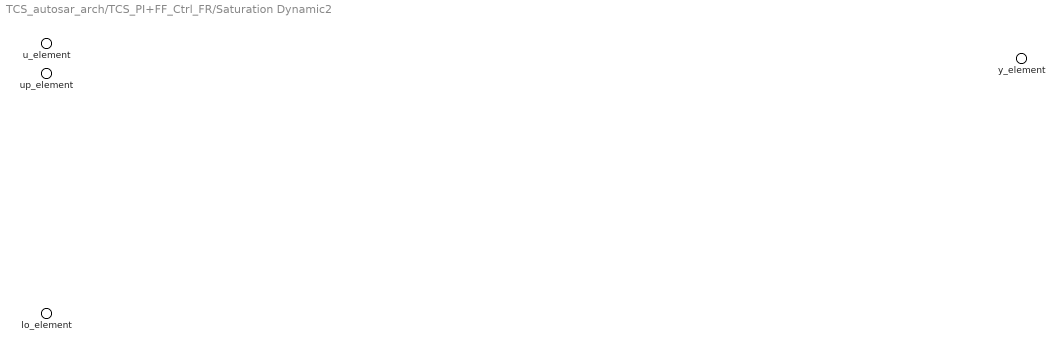
== system TCS_autosar_arch/TCS_PI+FF_Ctrl_FR/Saturation Dynamic2 ==
  up_element : Inport  PortName=up
  u_element : Inport  Port=2  PortName=u
  lo_element : Inport  Port=3  PortName=lo
  y_element : Outport  PortName=y

== system TCS_autosar_arch/TCS_PI+FF_Ctrl_R/Compare To Constant ==
  u_element : Inport  PortName=u
  y_element : Outport  PortName=y

== system TCS_autosar_arch/TCS_PI+FF_Ctrl_R/Compare To Constant1 ==
  u_element : Inport  PortName=u
  y_element : Outport  PortName=y

== system TCS_autosar_arch/TCS_PI+FF_Ctrl_R/Compare To Constant2 ==
  u_element : Inport  PortName=u
  y_element : Outport  PortName=y

== system TCS_autosar_arch/TCS_PI+FF_Ctrl_R/Compare To Zero ==
  u_element : Inport  PortName=u
  y_element : Outport  PortName=y

== system TCS_autosar_arch/TCS_PI+FF_Ctrl_R/Detect Rise Positive ==
  U_element : Inport  PortName=U
  Y_element : Outport  PortName=Y

== system TCS_autosar_arch/TCS_PI+FF_Ctrl_R/Latch_on ==
  Set_element : Inport  PortName=Set
  Reset_element : Inport  Port=2  PortName=Reset
  flg_TCSActv_element : Outport  PortName=flg_TCSActv

== system TCS_autosar_arch/TCS_PI+FF_Ctrl_R/RisingTimer ==
  Set_element : Inport  PortName=Set
  Timer_element : Inport  Port=2  PortName=Timer
  TCSExit_element : Outport  PortName=TCSExit

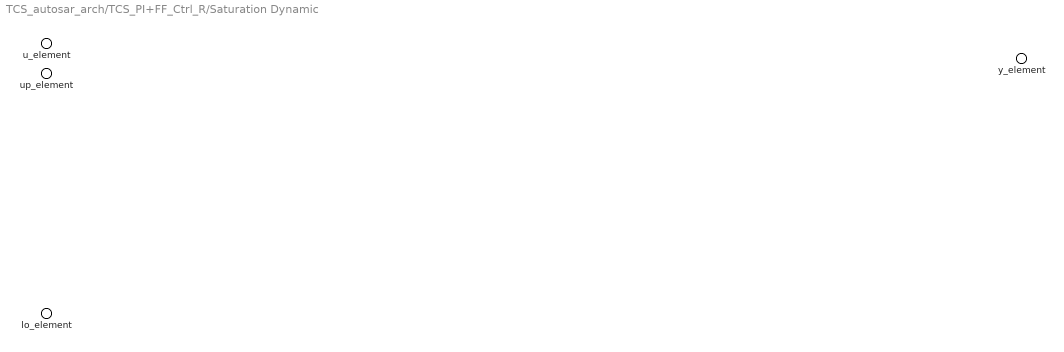
== system TCS_autosar_arch/TCS_PI+FF_Ctrl_R/Saturation Dynamic ==
  up_element : Inport  PortName=up
  u_element : Inport  Port=2  PortName=u
  lo_element : Inport  Port=3  PortName=lo
  y_element : Outport  PortName=y

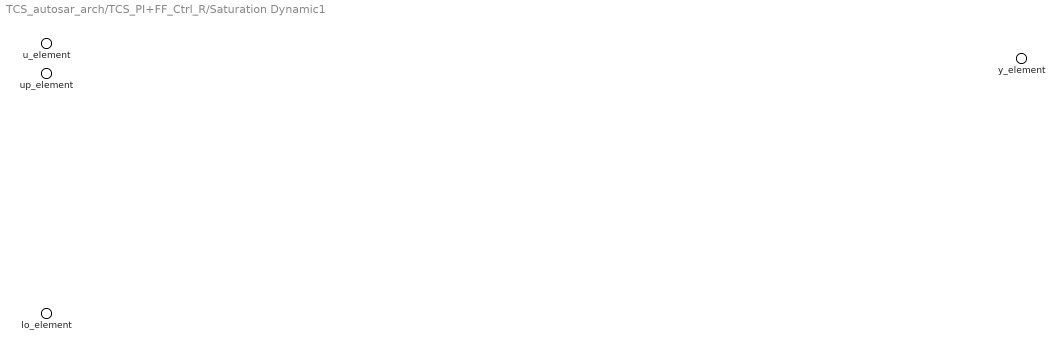
== system TCS_autosar_arch/TCS_PI+FF_Ctrl_R/Saturation Dynamic1 ==
  up_element : Inport  PortName=up
  u_element : Inport  Port=2  PortName=u
  lo_element : Inport  Port=3  PortName=lo
  y_element : Outport  PortName=y

== system TCS_autosar_arch/TCS_PI+FF_Ctrl_R/Saturation Dynamic2 ==
  up_element : Inport  PortName=up
  u_element : Inport  Port=2  PortName=u
  lo_element : Inport  Port=3  PortName=lo
  y_element : Outport  PortName=y
